simulink model "liquid_level_control"  (R2022a)
settings: Solver=ode45  StartTime=0.0  StopTime=100.0  MaxStep=0.01  MinStep=0.001  RelTol=1e-3  EnableMultiTasking=on
undefined symbols (not defined in the file): fis, g, hmax, hmin, Kflow, Kgate, sigbuilder_block, Stank
libraries: fuzblock x1
settings Model: Creator=Сергей  LastModifiedBy=clever0ne
settings SolverCC: AlgebraicLoopSolver=TrustRegion
settings DataIOCC: SaveFormat=Array  SignalLogging=off  DSMLogging=off  ReturnWorkspaceOutputs=off
settings OptimizationCC: LifeSpan=inf
settings DebuggingCC: UnconnectedInputMsg=warning  UnconnectedOutputMsg=warning  UnconnectedLineMsg=warning  AllowSymbolicDim=off  SFUnexpectedBacktrackingDiag=warning  SFNoUnconditionalDefaultTransitionDiag=warning  SFExecutionAtInitializationDiag=none  SFMachineParentedDataDiag=warning  ArithmeticOperatorsInVariantConditions=warning
settings ModelReferenceCC: PropagateSignalLabelsOutOfModel=off
settings SFSimCC: SimUseLocalCustomCode=off  CustomCodeUndefinedFunction=UseInterfaceOnly
settings RTWCC: RTWUseLocalCustomCode=off
settings CodeAppCC: StateflowObjectComments=on
settings GRTTargetCC: TargetLangStandard=C89/C90 (ANSI)
settings ConfigComp: CovMetricSettings=dw  CovSaveCumulativeToWorkspaceVar=on  CovSaveSingleToWorkspaceVar=on  CovExternalEMLEnable=off

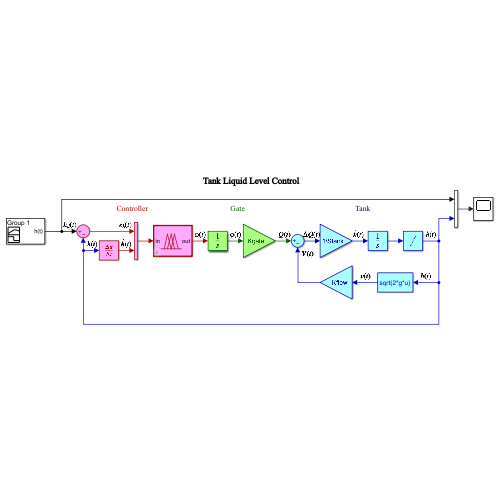
[thumbnail: Simulink's stored preview of the top-level diagram]
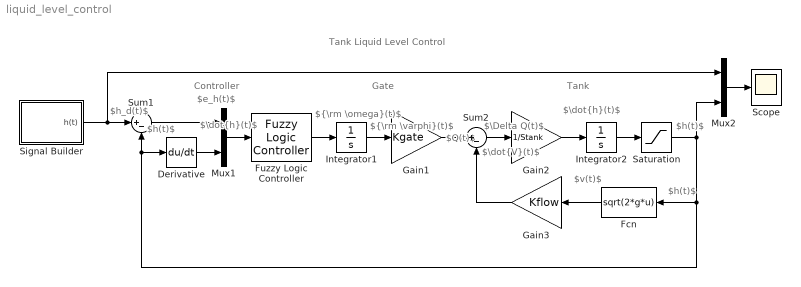
== system liquid_level_control ==
  note: $\dot{h}(t)$
  note: Tank
  note: Tank Liquid Level Control
  note: Controller
  note: Gate
  note: $e_h(t)$
  note: $h_d(t)$
  note: $h(t)$
  note: ${\rm \omega}(t)$
  note: ${\rm \varphi}(t)$
  note: $Q(t)$
  note: $\dot{V}(t)$
  note: $\Delta Q(t)$
  note: $\dot{h}(t)$
  note: $h(t)$
  note: $v(t)$
  note: $h(t)$
  Derivative : Derivative
  Fcn : Fcn  Expr=sqrt(2*g*u)
  Fuzzy Logic Controller : fuzblock/Fuzzy Logic  Controller  FIS=[fis]  OutputSampleNumber=101  DataType=double  FuzzifiedInputs=off  RuleFiringStrengths=off  RuleOutputs=off  AggregatedOutputs=off  SimulateUsing=Interpreted execution  OutOfRangeInputValueMessage=none  NoRuleFiredMessage=none  EmptyOutputFuzzySetMessage=none
  Gain1 : Gain  Gain=Kgate
  Gain2 : Gain  Gain=1/Stank
  Gain3 : Gain  Gain=Kflow
  Integrator1 : Integrator
  Integrator2 : Integrator
  Mux1 : Mux  Inputs=2
  Mux2 : Mux  Inputs=2
  Saturation : Saturate  UpperLimit=hmax  LowerLimit=hmin
  Scope : Scope
  Signal Builder : Subsystem  Tag=STV Subsys  LoadFcn=sigbuilder_block('load');  StartFcn=sigbuilder_block('start');  StopFcn=sigbuilder_block('stop');  ClipboardFcn=sigbuilder_block('clipboard');  mask(Sigbuilder block){tuvar=[0:10]}
      mask help: Simulink:masks:SigbuilderBlock_MD
      mask init:
      | if ~strcmp(get_param(bdroot(gcbh),'SimulationStatus'),'stopped') tuvar = sigbuilder_block('maskInit'); end
      settings: CopyFcn=sigbuilder_block('copy');  DeleteFcn=sigbuilder_block('delete');  ModelCloseFcn=sigbuilder_block('modelClose');  PreSaveFcn=sigbuilder_block('preSave');  PauseFcn=sigbuilder_block('pause');  ContinueFcn=sigbuilder_block('continue');  NameChangeFcn=sigbuilder_block('namechange');  OpenFcn=sigbuilder_block('open',[63.75 114.75 550.5 399.75 ]);  CloseFcn=sigbuilder_block('close');
      mask Display: plot(0, 0, 100, 100,[2, 2, 32, 32, 2], [68, 8, 8, 68, 68],[32, 2], [38, 38], [32, 19, 2],[53, 60, 44], [32, 17, 17, 2],[16, 16, 31, 31]);txt = getActiveGroup(gcbh);text(2, 100, txt,'verticalAlignment', 'top');
  Sum1 : Sum  Inputs=|+-
  Sum2 : Sum  Inputs=|+-
  wires:
  Gain2/1 -> Integrator2/1
  Sum2/1 -> Gain2/1
  Fcn/1 -> Gain3/1
  Gain3/1 -> Sum2/2
  Signal Builder/1(h(t)) -> Mux2/1, Sum1/1
  Mux1/1 -> Fuzzy Logic Controller/1
  Sum1/1 -> Mux1/1
  Derivative/1 -> Mux1/2
  Integrator2/1 -> Saturation/1
  Saturation/1 -> Mux2/2, Fcn/1, Derivative/1, Sum1/2
  Gain1/1 -> Sum2/1
  Integrator1/1 -> Gain1/1
  Fuzzy Logic Controller/1 -> Integrator1/1
  Mux2/1 -> Scope/1

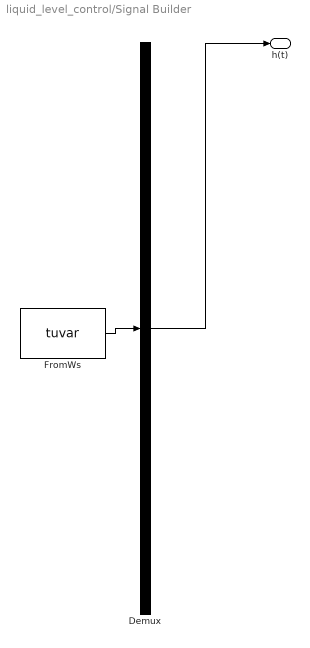
== system liquid_level_control/Signal Builder ==
  Demux : Demux  Tag=STV Demux  Outputs=1
      settings: DisplayOption=none
  FromWs : FromWorkspace  Tag=STV FromWs  VariableName=tuvar
      SigBuilderData=|
      | common.afterFinalStr = 'Extrapolate'
      | common.sampleTime = 0
      | dataSet.timeRange = [0 100]
      | dataSet.name = 'Group 1'
      | sbobj.Groups.Name = 'Group 1'
      | sbobj.Groups.Signals.Name = 'h(t)'
      | sbobj.Groups.Signals.XData = [0 1 1 60 60 100]
      | sbobj.Groups.Signals.YData = [0 0 1 1 0.4 0.4]
      | sbobj.Groups.TimeRange = [0 100]
  h(t) : Outport  Tag=STV Outport
  wires:
  Demux/1 -> h(t)/1
  FromWs/1 -> Demux/1
